simulink model "kf_test_1"  (R2018b)
settings: Solver=VariableStepAuto  StartTime=0.0  StopTime=60  RelTol=1e-3
values from neighbouring files (symbols this model uses):
  Rv = diag([10^-3 10^-3])    [KF_LQR_final.m]    (also in kf_test_1.m = 0; lab_init_lqr_hardware.m = diag([10^-5 10^-5]))
undefined symbols (not defined in the file or in its folder): Continuous, Time
libraries: cstblocks x8, ctrlSharedLib x1
settings Model: Creator=prana  LastModifiedBy=prana

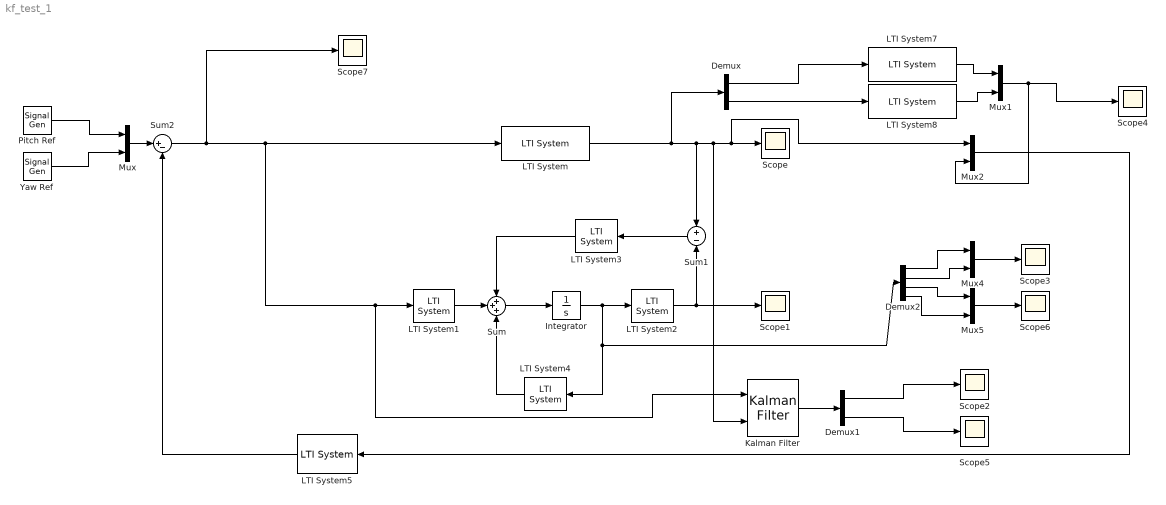
== system kf_test_1 ==
  Demux : Demux  Outputs=2
  Demux1 : Demux  Outputs=2
  Demux2 : Demux
  Integrator : Integrator
  Kalman Filter : ctrlSharedLib/Kalman Filter  TimeDomain=Continuous-Time  UseCurrentEstimator=on  ModelSource=LTI State-Space Variable  ModelSourceVariable=aero_sys  A=0.95  B=1  C=1  D=0  NumberOfStates=1  NumberOfInputs=1  NumberOfOutputs=1  InitialEstimateSource=Dialog  X0=0  P0=10  UseK=off  UseGH=off  NumberOfProcessNoiseInputs=1  G=1  TimeInvariantG=on  H=0  TimeInvariantH=on  Q=Rw  TimeInvariantQ=on  R=Rv  TimeInvariantR=on  N=0  TimeInvariantN=on  AddInputPort=on  AddEnablePort=off  OutputEstimatedY=off  OutputP=off  Ts=-1
      settings: SourceProductBaseCode=CT
  LTI System : cstblocks/LTI System  sys=aero_sys  IC=[]
  LTI System1 : cstblocks/LTI System  sys=B  IC=[]
  LTI System2 : cstblocks/LTI System  sys=C  IC=[]
  LTI System3 : cstblocks/LTI System  sys=Kf  IC=[]
  LTI System4 : cstblocks/LTI System  sys=A  IC=[]
  LTI System5 : cstblocks/LTI System  sys=K_lqr  IC=[]
  LTI System7 : cstblocks/LTI System  sys=Diff_LPF  IC=[]
  LTI System8 : cstblocks/LTI System  sys=Diff_LPF  IC=[]
  Mux{,1..2,4..5} (5 alike) : Mux  Inputs=2
  Pitch Ref : SignalGenerator  WaveForm=square  Amplitude=pi/6  Frequency=0.4  Units=rad/sec
  Scope{,1..7} (8 alike) : Scope
  Sum : Sum  Inputs=+++
  Sum1 : Sum  Inputs=+|-
  Sum2 : Sum  Inputs=|+-
  Yaw Ref : SignalGenerator  WaveForm=square  Amplitude=pi/4  Frequency=0.5  Units=rad/sec
  wires:
  LTI System/1 -> Demux/1, Kalman Filter/2, Mux2/1, Scope/1, Sum1/1
  LTI System2/1 -> Scope1/1, Sum1/2
  Sum1/1 -> LTI System3/1
  LTI System3/1 -> Sum/1
  LTI System1/1 -> Sum/2
  Sum/1 -> Integrator/1
  LTI System4/1 -> Sum/3
  Pitch Ref/1 -> Mux/1
  Yaw Ref/1 -> Mux/2
  Mux/1 -> Sum2/1
  LTI System5/1 -> Sum2/2
  Sum2/1 -> Scope7/1, Kalman Filter/1, LTI System1/1, LTI System/1
  LTI System7/1 -> Mux1/1
  Demux/2 -> LTI System8/1
  Demux/1 -> LTI System7/1
  LTI System8/1 -> Mux1/2
  Mux1/1 -> Mux2/2, Scope4/1
  Mux5/1 -> Scope6/1
  Mux4/1 -> Scope3/1
  Demux2/4 -> Mux5/2
  Demux2/3 -> Mux5/1
  Demux2/2 -> Mux4/2
  Demux2/1 -> Mux4/1
  Integrator/1 -> LTI System4/1, Demux2/1, LTI System2/1
  Kalman Filter/1 -> Demux1/1
  Demux1/1 -> Scope2/1
  Demux1/2 -> Scope5/1
  Mux2/1 -> LTI System5/1
